simulink model "Modello_definitivo"  (Simulink 9.2)
settings: Solver=ode45  StartTime=0*24*3600  StopTime=365*24*3600  MaxStep=3600  RelTol=1e-3  SampleTimeConstraint=Specified  EnableMultiTasking=on
undefined symbols (not defined in the file or in its folder): T_s_in
libraries: simulink x1
(part 2 of 2)

== system Modello_definitivo/Solar thermal storage/Lower part 3/Qgain/Controller Qgain/If Action Subsystem ==
  Action Port : ActionPort  ActionType=then
  J to MJ : Constant  Value=0
  Out1 : Outport
  wires:
  J to MJ/1 -> Out1/1

== system Modello_definitivo/Solar thermal storage/Lower part 3/Qgain/Controller Qgain/If Action Subsystem1 ==
  In1 : Inport
  Action Port : ActionPort  ActionType=elseif
  Out1 : Outport
  wires:
  In1/1 -> Out1/1

== system Modello_definitivo/Solar thermal storage/Lower part 3/Qgain/Controller Qgain/If Action Subsystem3 ==
  In1 : Inport
  Action Port : ActionPort  ActionType=elseif
  Out1 : Outport
  wires:
  In1/1 -> Out1/1

== system Modello_definitivo/Solar thermal storage/Lower part 3/Qgain/Controller Qgain/Qstored ==
  Add2 : Sum  Inputs=-+
  Product3 : Product  Inputs=***  SaturateOnIntegerOverflow=on  OutDataTypeStr=Inherit: Same as first input
  Qstored : Outport
  wires:
  Product3/1 -> Qstored/1
  [T_acq] -> Add2/1
  [T3] -> Add2/2
  Add2/1 -> Product3/1
  [m] -> Product3/2
  [Cp_water] -> Product3/3
